simulink model "Battery_Model"  (R2018a)
settings: Solver=VariableStepAuto  StartTime=0.0  StopTime=101  RelTol=1e-3
values from neighbouring files (symbols this model uses):
  Charge_Flag = 1    [Prj_5_BatteryModel.m]
  CN = 2.3*100    (= 230)    [Prj_5_BatteryModel.m]
  I = 2.3    [Prj_5_BatteryModel.m]
  OCV = data(:,2)    [Prj_5_BatteryModel.m]
  R_charge = data(:,3)    [Prj_5_BatteryModel.m]
  R_discharge = data(:,4)    [Prj_5_BatteryModel.m]
  SOC = data(:,1)    [Prj_5_BatteryModel.m]
settings Model: Creator=Dpt_Mas  LastModifiedBy=Dpt_Mas

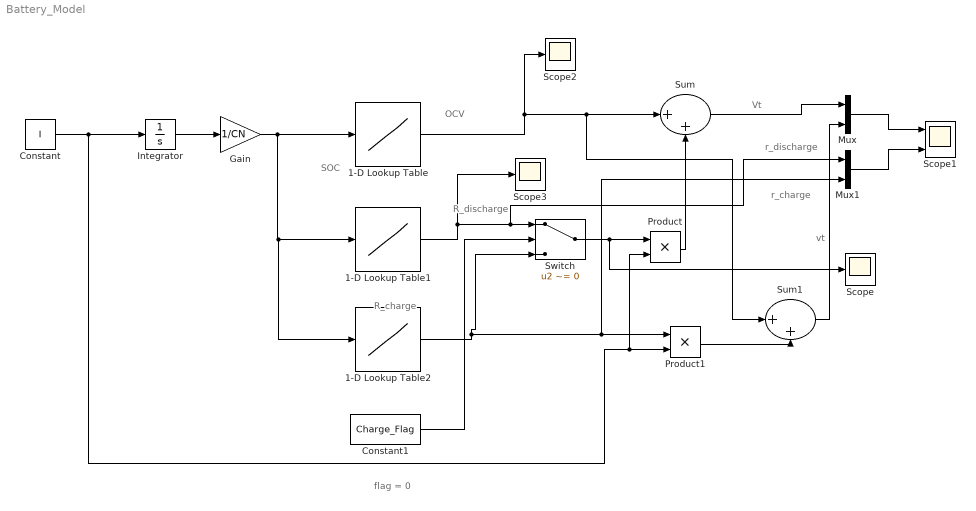
== system Battery_Model ==
  note: r_charge
  note: r_discharge
  note: vt
  note: flag = 0
  note: R_charge
  note: Vt
  note: R_discharge
  note: OCV
  note: SOC
  1-D Lookup Table : Lookup_n-D  NumberOfTableDimensions=1  BreakpointsForDimension1=SOC  Table=OCV  InternalRulePriority=Speed  RndMeth=Simplest  InputSameDT=on
  1-D Lookup Table1 : Lookup_n-D  NumberOfTableDimensions=1  BreakpointsForDimension1=SOC  Table=R_discharge  InternalRulePriority=Speed  RndMeth=Simplest  InputSameDT=on
  1-D Lookup Table2 : Lookup_n-D  NumberOfTableDimensions=1  BreakpointsForDimension1=SOC  Table=R_charge  InternalRulePriority=Speed  RndMeth=Simplest  InputSameDT=on
  Constant : Constant  Value=I
  Constant1 : Constant  Value=Charge_Flag  OutDataTypeStr=uint8
  Gain : Gain  Gain=1/CN
  Integrator : Integrator
  Mux : Mux  Inputs=2
  Mux1 : Mux  Inputs=2
  Product : Product
  Product1 : Product
  Scope : Scope
  Scope1 : Scope  NumInputPorts=2
  Scope2 : Scope
  Scope3 : Scope
  Sum : Sum  Inputs=|++
  Sum1 : Sum  Inputs=|++
  Switch : Switch  Criteria=u2 ~= 0
  wires:
  Integrator/1 -> Gain/1
  1-D Lookup Table1/1 -> Scope3/1, Mux1/1, Switch/1
  Constant/1 -> Product1/2, Product/2, Integrator/1
  1-D Lookup Table/1 -> Scope2/1, Sum1/1, Sum/1
  Product/1 -> Sum/2
  Switch/1 -> Scope/1, Product/1
  1-D Lookup Table2/1 -> Switch/3, Product1/1, Mux1/2
  Gain/1 -> 1-D Lookup Table2/1, 1-D Lookup Table1/1, 1-D Lookup Table/1
  Constant1/1 -> Switch/2
  Product1/1 -> Sum1/2
  Mux/1 -> Scope1/1
  Sum1/1 -> Mux/2
  Mux1/1 -> Scope1/2
  Sum/1 -> Mux/1
